simulink model "MPC"  (R2026a)
settings: Solver=VariableStepAuto  StopTime=15
values from neighbouring files (symbols this model uses):
  A = [0 0 1 0; 0 0 0 1; -2.517 0 -10.915 0; 0 0 0 0]    [sistema_lineare.m]
  B = [0 0; 0 0; 21.83 0; 0 1.236]    [sistema_lineare.m]
  C = [1 0 0 0; 0 1 0 0; 0 0 1 0; 0 0 0 1]    [sistema_lineare.m]
  D = [0 0; 0 0; 0 0; 0 0]    [sistema_lineare.m]
libraries: mpclib x2, simulink x1
settings Model: Creator=user  LastModifiedBy=user

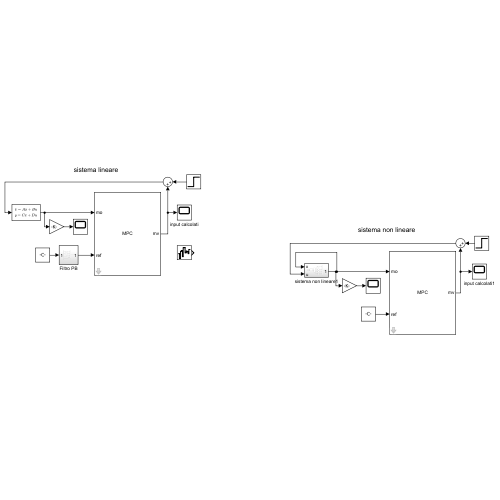
[thumbnail: Simulink's stored preview of the top-level diagram]
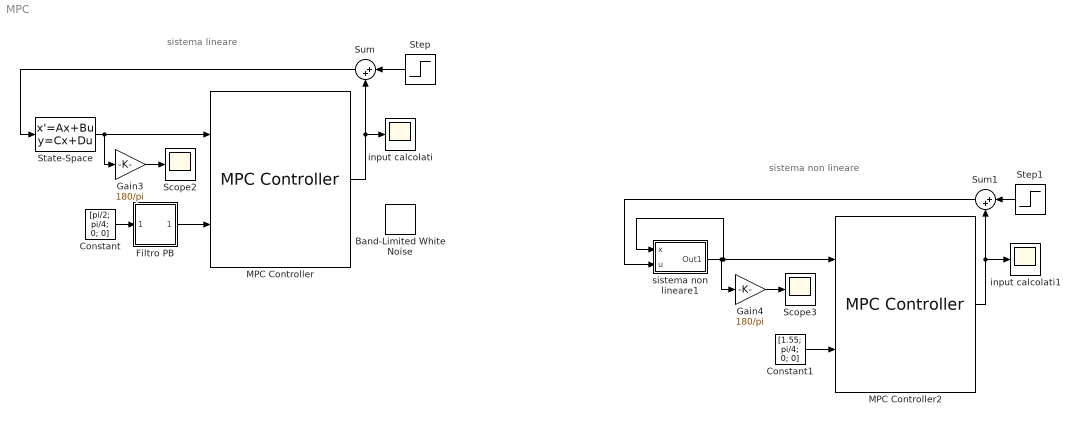
== system MPC ==
  note: sistema non lineare
  note: sistema lineare
  Band-Limited White Noise : simulink/Sources/Band-Limited White Noise  Cov=[0.001]  Ts=0.1  seed=[23341]
  Constant : Constant  Value=[pi/2; pi/4; 0; 0]
  Constant1 : Constant  Value=[1.55; pi/4; 0; 0]
  Filtro PB : Subsystem
  Gain3 : Gain  Gain=180/pi
  Gain4 : Gain  Gain=180/pi
  MPC Controller : mpclib/MPC Controller  SCDEnableBlockLinearizationSpecification=on  mpcobj=mpc_obj  x0=mstate  is_multiple=0  enable_value=0  return_u0=off  updateMPCinCallerWorkspace=on  md_inport=off  mv_inport=off  uref_inport=off  return_cost=off  return_mvseq=off  return_qpstatus=off  return_xseq=off  return_state=off  return_ovseq=off  state_inport=off  umin_inport=off  umax_inport=off  ymin_inport=off  ymax_inport=off  cc_inport=off  ywt_inport=off  uwt_inport=off  duwt_inport=off  rhoeps_inport=off  pm_inport=off  MaximumP=10  HorizonChoice=FixedHorizon  n_ts=0.05  n_p=30  n_mv=2  n_md=0  n_ud=2  n_mo=4  n_uo=0  BlockDataType=double  SampleTimeInherited=off  switch_inport=off
  MPC Controller2 : mpclib/MPC Controller  SCDEnableBlockLinearizationSpecification=on  mpcobj=mpc_obj  x0=mstate  is_multiple=0  enable_value=0  return_u0=off  updateMPCinCallerWorkspace=on  md_inport=off  mv_inport=off  uref_inport=off  return_cost=off  return_mvseq=off  return_qpstatus=off  return_xseq=off  return_state=off  return_ovseq=off  state_inport=off  umin_inport=off  umax_inport=off  ymin_inport=off  ymax_inport=off  cc_inport=off  ywt_inport=off  uwt_inport=off  duwt_inport=off  rhoeps_inport=off  pm_inport=off  MaximumP=10  HorizonChoice=FixedHorizon  n_ts=0.05  n_p=30  n_mv=2  n_md=0  n_ud=2  n_mo=4  n_uo=0  BlockDataType=double  SampleTimeInherited=off  switch_inport=off
  Scope2 : Scope
      settings: Title=sistema lineare  ActiveDisplayYMinimum=-140.81513278336831  ActiveDisplayYMaximum=709.77673126109755  YLabel=dinamiche stati  DataLoggingVariableName=ScopeData2
  Scope3 : Scope
      settings: Title=sistema non lineare  ActiveDisplayYMinimum=-19.397001262726704  ActiveDisplayYMaximum=121.42315409925638  YLabel=dinamiche stati  DataLoggingVariableName=ScopeData4
  State-Space : StateSpace  A=A  B=B  C=C  D=D  InitialCondition=[0.117; 0; 0; 0]
  Step : Step  Time=5  SampleTime=0
  Step1 : Step  Time=5  FinalValue=0.1  SampleTime=0
  Sum : Sum  Inputs=|++
  Sum1 : Sum  Inputs=|++
  input calcolati : Scope
      settings: Title=ingressi  ActiveDisplayYMinimum=-4.0742093297714348  ActiveDisplayYMaximum=3.4693159947526597  DataLoggingVariableName=ScopeData3
  input calcolati1 : Scope
      settings: Title=ingressi  ActiveDisplayYMinimum=-1  ActiveDisplayYMaximum=1  DataLoggingVariableName=ScopeData5
  sistema non lineare1 : Subsystem
  wires:
  Sum/1 -> State-Space/1
  MPC Controller/1 -> Sum/2, input calcolati/1
  Gain3/1 -> Scope2/1
  sistema non lineare1/1(Out1) -> MPC Controller2/1, sistema non lineare1/1(x), Gain4/1
  MPC Controller2/1 -> input calcolati1/1, Sum1/2
  Gain4/1 -> Scope3/1
  Sum1/1 -> sistema non lineare1/2(u)
  State-Space/1 -> Gain3/1, MPC Controller/1
  Constant1/1 -> MPC Controller2/2
  Step1/1 -> Sum1/1
  Constant/1 -> Filtro PB/1(In1)
  Filtro PB/1(Out1) -> MPC Controller/2
  Step/1 -> Sum/1

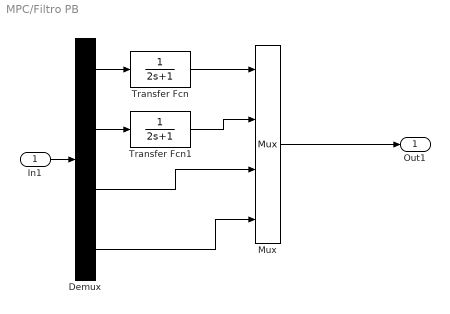
== system MPC/Filtro PB ==
  In1 : Inport
  Demux : Demux
  Mux : Mux
  Transfer Fcn : TransferFcn  Denominator=[2 1]
  Transfer Fcn1 : TransferFcn  Denominator=[2 1]
  Out1 : Outport
  wires:
  In1/1 -> Demux/1
  Demux/1 -> Transfer Fcn/1
  Demux/2 -> Transfer Fcn1/1
  Transfer Fcn/1 -> Mux/1
  Transfer Fcn1/1 -> Mux/2
  Demux/3 -> Mux/3
  Demux/4 -> Mux/4
  Mux/1 -> Out1/1

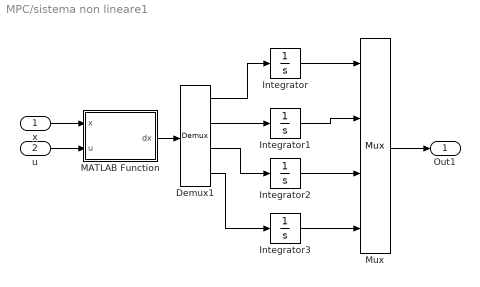
== system MPC/sistema non lineare1 ==
  x : Inport
  u : Inport  Port=2
  Demux1 : Demux
  Integrator : Integrator  InitialCondition=1.55
  Integrator1 : Integrator  InitialCondition=pi/4
  Integrator2 : Integrator
  Integrator3 : Integrator
  MATLAB Function : MATLAB Function  TreatAsAtomicUnit=on
  Mux : Mux
  Out1 : Outport  PortDimensions=4
  wires:
  MATLAB Function/1(dx) -> Demux1/1
  Demux1/1 -> Integrator/1
  Demux1/2 -> Integrator1/1
  Mux/1 -> Out1/1
  x/1 -> MATLAB Function/1(x)
  u/1 -> MATLAB Function/2(u)
  Integrator/1 -> Mux/1
  Integrator1/1 -> Mux/2
  Integrator3/1 -> Mux/4
  Integrator2/1 -> Mux/3
  Demux1/3 -> Integrator2/1
  Demux1/4 -> Integrator3/1

== matlab function MPC/sistema non lineare1/MATLAB Function ==
  data: x input; u input; dx output
function dx = trms_dynamics(x, u)
    % Estrazione degli stati dal vettore x
    x1 = x(1);
    x2 = x(2);
    x3 = x(3);
    x4 = x(4);
    
    % Estrazione degli ingressi dal vettore u
    u1 = u(1);
    u2 = u(2);
    
    % Calcolo delle equazioni differenziali
    dx1 = x3;
    dx2 = x4;
    
    % Dinamica di x3
    dx3 = 21.83 * (0.0981*cos(x1) - 0.833*sin(x1) + u1 - 0.195*(x4^2)*sin(x1)*cos(x1) - 0.5*x3);
    
    % Dinamica di x4 (divisa in numeratore e denominatore per chiarezza)
    num_dx4 = u2*cos(x1) - 0.01*x4;
    den_dx4 = 0.01667*(sin(x1)^2) + 0.03728*(cos(x1)^2) + 0.00015;
    dx4 = num_dx4 / den_dx4;
    
    % Vettore colonna delle derivate
    dx = [dx1; dx2; dx3; dx4];
end
